simulink model "model"  (R2015b)
settings: Solver=VariableStepAuto  StartTime=0.0  StopTime=10.0  RelTol=1e-3
settings Model: Creator=Pepe  LastModifiedBy=Pepe

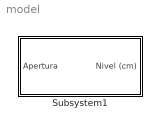
== system model ==
  Subsystem1 : Subsystem

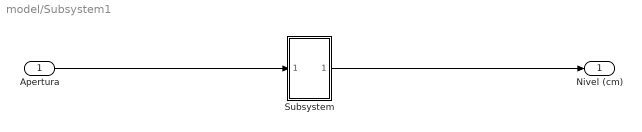
== system model/Subsystem1 ==
  Apertura : Inport
  Subsystem : Subsystem
  Nivel (cm) : Outport
  wires:
  Subsystem/1(Out1) -> Nivel (cm)/1
  Apertura/1 -> Subsystem/1(In1)

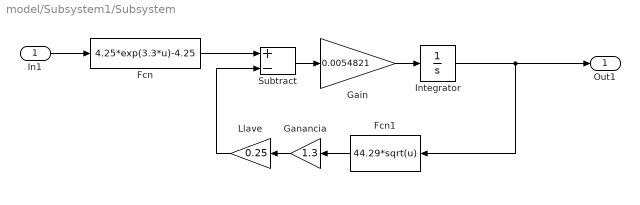
== system model/Subsystem1/Subsystem ==
  In1 : Inport
  Fcn : Fcn  Expr=4.25*exp(3.3*u)-4.25
  Fcn1 : Fcn  Expr=44.29*sqrt(u)
  Gain : Gain  Gain=0.0054821
  Ganancia : Gain  Gain=1.3
  Integrator : Integrator  InitialCondition=15  LimitOutput=on  UpperSaturationLimit=78  LowerSaturationLimit=0
  Llave : Gain  Gain=0.25
  Subtract : Sum  Inputs=+-
  Out1 : Outport
  wires:
  Llave/1 -> Subtract/2
  Fcn1/1 -> Ganancia/1
  Gain/1 -> Integrator/1
  Fcn/1 -> Subtract/1
  Ganancia/1 -> Llave/1
  Subtract/1 -> Gain/1
  In1/1 -> Fcn/1
  Integrator/1 -> Out1/1, Fcn1/1
